simulink model "Sorting"  (R2025b)
settings: Solver=VariableStepAuto  StartTime=0.0  StopTime=10.0  RelTol=1e-3
libraries: opcualib x1
settings Model: Creator=guilh  LastModifiedBy=guilh

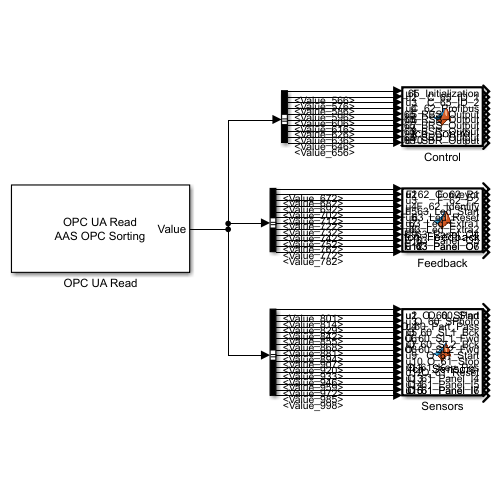
[thumbnail: Simulink's stored preview of the top-level diagram]
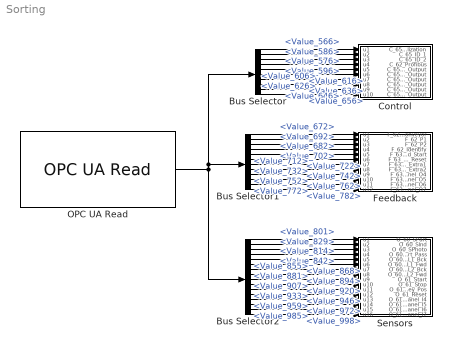
== system Sorting ==
  Bus Selector : BusSelector  OutputSignals=Value_566,Value_576,Value_586,Value_596,Value_606,Value_616,Value_626,Value_636,Value_646,Value_656
  Bus Selector1 : BusSelector  OutputSignals=Value_672,Value_682,Value_692,Value_702,Value_712,Value_722,Value_732,Value_742,Value_752,Value_762,Value_772,Value_782
  Bus Selector2 : BusSelector  OutputSignals=Value_801,Value_814,Value_829,Value_842,Value_855,Value_868,Value_881,Value_894,Value_907,Value_920,Value_933,Value_946,Value_959,Value_972,Value_985,Value_998
  Control : MATLAB Function  TreatAsAtomicUnit=on
  Feedback : MATLAB Function  TreatAsAtomicUnit=on
  OPC UA Read : opcualib/OPC UA Read  SelectedServer=AAS OPC Sorting  ServerList=AAS OPC Sorting  NodeList={ '1', 'Value', '6', '566', '1'; '2', 'Value', '6', '576', '1'; '3', 'Value', '6', '586', '1'; '4', 'Value', '6', '596', '1'; '5', 'Value', '6', '606', '1'; '6', 'Value', '6', '616', '1'; '7', 'Value', '6', '626', '1'; '8', 'Value', '6', '636', '1'; '9', 'Value', '6', '646', '1'; '10', 'Value', '6', '656', '1'; '11', 'Value', '6', '672', '1'; '12', 'Value', '6', '682', '1'; '13', 'Value', '6', '692', '1'; '14', 'Value', '6', '702', '1'; '15', 'Value', '6', '712', '1'; '16', 'Value', '6', '722', '1'; '17', 'Value', '6', '732', '1'; '18', 'Value', '6', '742', '1'; '19', 'Value', '6', '752', '1'; '20', 'Value', '6', '762', '1'; '21', 'Value', '6', '772', '1'; '22', 'Value', '6', '782', '1'; '23', 'Value', '6', '801', '1'; '24', 'Value', '6', '814', '1'; '25', 'Value', '6', '829', '1'; '26', 'Value', '6', '842', '1'; '27', 'Value', '6', '855', '1'; '28', 'Value', '6', '868', '1'; '29', 'Value', '6', '881', '1'; '30', 'Value', '6', '894', '1'; '31', 'Value', '6', '907', '1'; '32', 'Value', '6', '920', '1'; '33', 'Value', '6', '933', '1'; '34', 'Value', '6', '946', '1'; '35', 'Value', '6', '959', '1'; '36', 'Value', '6', '972', '1'; '37', 'Value', '6', '985', '1'; '38', 'Value', '6', '998', '1' }  ShowQualityPort=off  ShowTimestampPort=off  ShowTimestampPortAs=Seconds since start  SampleTime=-1
  Sensors : MATLAB Function  TreatAsAtomicUnit=on
  wires:
  OPC UA Read/1 -> Bus Selector2/1, Bus Selector/1, Bus Selector1/1
  Bus Selector/1 -> Control/1(u1)  "<Value_566>"
  Bus Selector/2 -> Control/2(u2)  "<Value_576>"
  Bus Selector/3 -> Control/3(u3)  "<Value_586>"
  Bus Selector/4 -> Control/4(u4)  "<Value_596>"
  Bus Selector/5 -> Control/5(u5)  "<Value_606>"
  Bus Selector/6 -> Control/6(u6)  "<Value_616>"
  Bus Selector/7 -> Control/7(u7)  "<Value_626>"
  Bus Selector/8 -> Control/8(u8)  "<Value_636>"
  Bus Selector/9 -> Control/9(u9)  "<Value_646>"
  Bus Selector/10 -> Control/10(u10)  "<Value_656>"
  Bus Selector1/1 -> Feedback/1(u1)  "<Value_672>"
  Bus Selector1/2 -> Feedback/2(u2)  "<Value_682>"
  Bus Selector1/3 -> Feedback/3(u3)  "<Value_692>"
  Bus Selector1/4 -> Feedback/4(u4)  "<Value_702>"
  Bus Selector1/5 -> Feedback/5(u5)  "<Value_712>"
  Bus Selector1/6 -> Feedback/6(u6)  "<Value_722>"
  Bus Selector1/7 -> Feedback/7(u7)  "<Value_732>"
  Bus Selector1/8 -> Feedback/8(u8)  "<Value_742>"
  Bus Selector1/9 -> Feedback/9(u9)  "<Value_752>"
  Bus Selector1/10 -> Feedback/10(u10)  "<Value_762>"
  Bus Selector1/11 -> Feedback/11(u11)  "<Value_772>"
  Bus Selector1/12 -> Feedback/12(u12)  "<Value_782>"
  Bus Selector2/1 -> Sensors/1(u1)  "<Value_801>"
  Bus Selector2/2 -> Sensors/2(u2)  "<Value_814>"
  Bus Selector2/3 -> Sensors/3(u3)  "<Value_829>"
  Bus Selector2/4 -> Sensors/4(u4)  "<Value_842>"
  Bus Selector2/5 -> Sensors/5(u5)  "<Value_855>"
  Bus Selector2/6 -> Sensors/6(u6)  "<Value_868>"
  Bus Selector2/7 -> Sensors/7(u7)  "<Value_881>"
  Bus Selector2/8 -> Sensors/8(u8)  "<Value_894>"
  Bus Selector2/9 -> Sensors/9(u9)  "<Value_907>"
  Bus Selector2/10 -> Sensors/10(u10)  "<Value_920>"
  Bus Selector2/11 -> Sensors/11(u11)  "<Value_933>"
  Bus Selector2/12 -> Sensors/12(u12)  "<Value_946>"
  Bus Selector2/13 -> Sensors/13(u13)  "<Value_959>"
  Bus Selector2/14 -> Sensors/14(u14)  "<Value_972>"
  Bus Selector2/15 -> Sensors/15(u15)  "<Value_985>"
  Bus Selector2/16 -> Sensors/16(u16)  "<Value_998>"

== matlab function Sorting/Control ==
  data: u1 input; C_65_Initialization output; u2 input; u3 input; u4 input; u5 input; u6 input; u7 input; u8 input; u9 input; u10 input; C_65_ID_1 output; C_65_ID_2 output; C_62_Profibus output; C_65_RBS_Output output; C_65_RSB_Output output; C_65_BRS_Output output; C_65_BSR_Output output; C_65_SRB_Output output; C_65_SBR_Output output
function [C_65_Initialization, C_65_ID_1, C_65_ID_2, ...
          C_62_Profibus,C_65_RBS_Output, C_65_RSB_Output, ...
          C_65_BRS_Output, C_65_BSR_Output,C_65_SRB_Output,... 
          C_65_SBR_Output] = ...
          fcn_Control(u1,u2,u3,u4,u5,u6,u7,u8,u9,u10)

    C_65_Initialization = u1;
    C_65_ID_1           = u2;
    C_65_ID_2           = u3;
    C_62_Profibus       = u4;
    C_65_RBS_Output     = u5;
    C_65_RSB_Output     = u6;
    C_65_BRS_Output     = u7;
    C_65_BSR_Output     = u8;
    C_65_SRB_Output     = u9;
    C_65_SBR_Output     = u10;

== matlab function Sorting/Feedback ==
  data: u1 input; F_62_Conveyor output; u2 input; u3 input; u4 input; u5 input; u6 input; u7 input; u8 input; u9 input; u10 input; u11 input; u12 input; F_62_P1 output; F_62_P2 output; F_62_Identify output; F_63_Led_Start output; F_63_Led_Reset output; F_63_Led_Extra1 output; F_63_Led_Extra2 output; F_63_Panel_O4 output; F_63_Panel_O5 output; F_63_Panel_O6 output; F_63_Panel_O7 output
function [F_62_Conveyor, F_62_P1, F_62_P2, F_62_Identify, ...
          F_63_Led_Start, F_63_Led_Reset, F_63_Led_Extra1, F_63_Led_Extra2, ...
          F_63_Panel_O4, F_63_Panel_O5, F_63_Panel_O6, F_63_Panel_O7] = ...
          fcn_Feedback(u1,u2,u3,u4,u5,u6,u7,u8,u9,u10,u11,u12)

    F_62_Conveyor   = u1;
    F_62_P1         = u2;
    F_62_P2         = u3;
    F_62_Identify   = u4;

    F_63_Led_Start  = u5;
    F_63_Led_Reset  = u6;
    F_63_Led_Extra1 = u7;
    F_63_Led_Extra2 = u8;

    F_63_Panel_O4   = u9;
    F_63_Panel_O5   = u10;
    F_63_Panel_O6   = u11;
    F_63_Panel_O7   = u12;

== matlab function Sorting/Sensors ==
  data: u1 input; O_60_SPart output; u2 input; u3 input; u4 input; u5 input; u6 input; u7 input; u8 input; u9 input; u10 input; u11 input; u12 input; u13 input; u14 input; u15 input; u16 input; O_60_Slnd output; O_60_SPhoto output; O_60_Part_Pass output; O_60_SL1_Bck output; O_60_SL1_Fwd output; O_60_SL2_Bck output; O_60_SL2_Fwd output; O_61_Start output; O_61_Stop output; O_61_Key_Pos output; O_61_Reset output; O_61_Panel_I4 output; O_61_Panel_I5 output; O_61_Panel_I6 output; O_61_Panel_I7 output
function [ ...
    O_60_SPart, O_60_Slnd, O_60_SPhoto, O_60_Part_Pass, ...
    O_60_SL1_Bck, O_60_SL1_Fwd, O_60_SL2_Bck, O_60_SL2_Fwd, ...
    O_61_Start, O_61_Stop, O_61_Key_Pos, O_61_Reset, ...
    O_61_Panel_I4, O_61_Panel_I5, O_61_Panel_I6, O_61_Panel_I7] = ...
    fcn_Sensors(u1,u2,u3,u4,u5,u6,u7,u8,u9,u10,u11,u12,u13,u14,u15,u16)

O_60_SPart      = u1;
O_60_Slnd       = u2;
O_60_SPhoto     = u3;
O_60_Part_Pass  = u4;

O_60_SL1_Bck    = u5;
O_60_SL1_Fwd    = u6;
O_60_SL2_Bck    = u7;
O_60_SL2_Fwd    = u8;

O_61_Start      = u9;
O_61_Stop       = u10;
O_61_Key_Pos    = u11;
O_61_Reset      = u12;

O_61_Panel_I4   = u13;
O_61_Panel_I5   = u14;
O_61_Panel_I6   = u15;
O_61_Panel_I7   = u16;
